simulink model "ultimul_ex"  (R2020a)
settings: Solver=VariableStepAuto  StartTime=0.0  StopTime=500  RelTol=1e-3
values from neighbouring files (symbols this model uses):
  Te = 0.6    [datewinpim - Copy.m]    (also in proces_etapa1.m = 2.5; proces_etapa2.m = 2.5; script3.m; script4.m)
settings Model: Creator=user  LastModifiedBy=user

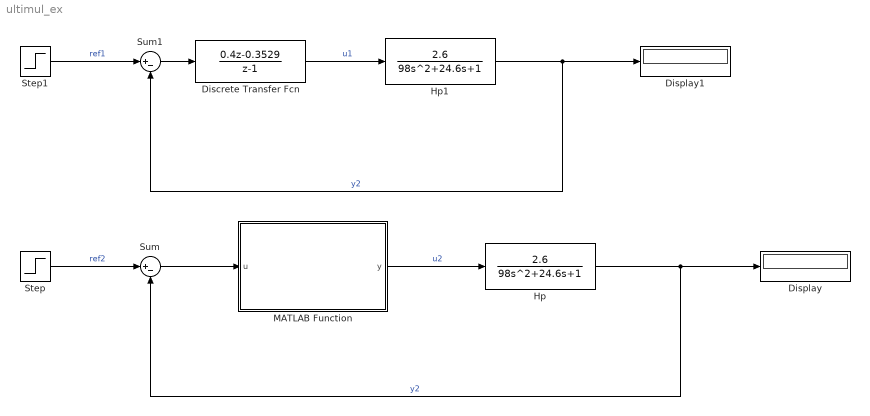
== system ultimul_ex ==
  Discrete Transfer Fcn : DiscreteTransferFcn  Numerator=[0.4 -0.3529]  Denominator=[1 -1]  SampleTime=2.5
  Display : Display
  Display1 : Display
  Hp : TransferFcn  Numerator=[2.6]  Denominator=[98 24.6 1]
  Hp1 : TransferFcn  Numerator=[2.6]  Denominator=[98 24.6 1]
  MATLAB Function : MATLAB Function  TreatAsAtomicUnit=on
  Step : Step  Time=0  SampleTime=Te
  Step1 : Step  Time=0  SampleTime=Te
  Sum : Sum  Inputs=|+-
  Sum1 : Sum  Inputs=|+-
  wires:
  Hp/1 -> Display/1, Sum/2  "y2"
  Step/1 -> Sum/1  "ref2"
  MATLAB Function/1(y) -> Hp/1  "u2"
  Sum/1 -> MATLAB Function/1(u)
  Discrete Transfer Fcn/1 -> Hp1/1  "u1"
  Hp1/1 -> Display1/1, Sum1/2  "y2"
  Step1/1 -> Sum1/1  "ref1"
  Sum1/1 -> Discrete Transfer Fcn/1

== matlab function ultimul_ex/MATLAB Function ==
  settings: updateMethod=DISCRETE
  data: u input; y output
function y = fcn(u)

persistent s

if isempty(s)
    s = u;
end

Kpi = 0.98/2.6;
Ti = 19.6;

u_k = Kpi*(1 + 1/(Ti*s));
 %scalam iesirea

u_s = u_k/1.03; 
 
y = u_s;
